simulink model "OPC_UA_daniel"  (R2024b)
settings: Solver=FixedStepAuto  StartTime=0.0  StopTime=inf  FixedStep=0.01  RelTol=1e-3
libraries: opcualib x1
settings Model: Creator=Are-Laptop  LastModifiedBy=Are-Laptop

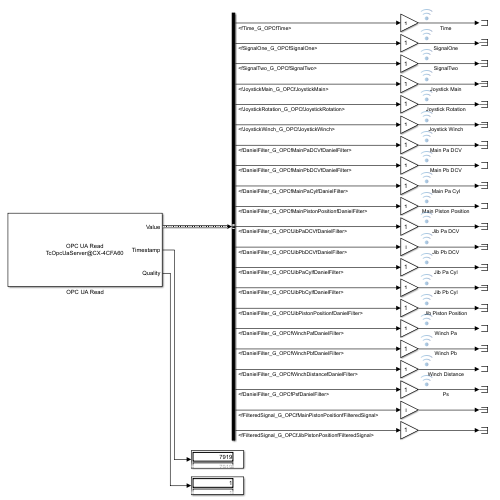
[thumbnail: Simulink's stored preview of the top-level diagram]
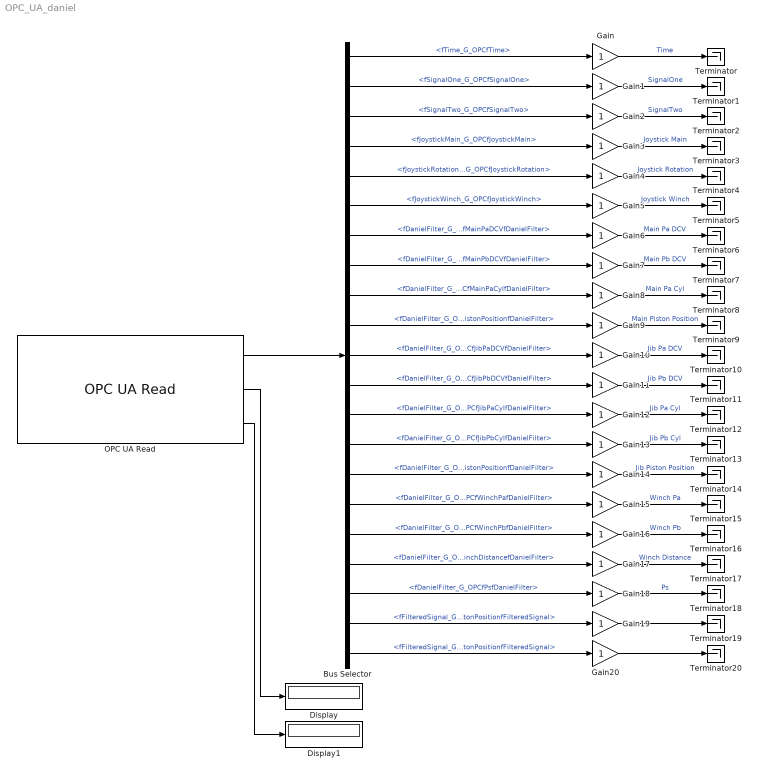
== system OPC_UA_daniel ==
  Bus Selector : BusSelector  OutputSignals=fTime_G_OPCfTime,fSignalOne_G_OPCfSignalOne,fSignalTwo_G_OPCfSignalTwo,fJoystickMain_G_OPCfJoystickMain,fJoystickRotation_G_OPCfJoystickRotation,fJoystickWinch_G_OPCfJoystickWinch,fDanielFilter_G_OPCfMainPaDCVfDanielFilter,fDanielFilter_G_OPCfMainPbDCVfDanielFilter,fDanielFilter_G_OPCfMainPaCylfDanielFilter,fDanielFilter_G_OPCfMainPistonPositionfDanielFilter,fDanielFilter_G_OPCfJibPaDCVfDanielFilter,fDanielFilter_G_OPCfJibPbDCVfDanielFilter,fDanielFilter_G_OPCfJibPaCylfDanielFilter,fDanielFilter_G_OPCfJibPbCylfDanielFilter,fDanielFilter_G_OPCfJibPistonPositionfDanielFilter,fDanielFilter_G_OPCfWinchPafDanielFilter,fDanielFilter_G_OPCfWinchPbfDanielFilter,fDanielFilter_G_OPCfWinchDistancefDanielFilter,fDanielFilter_G_OPCfPsfDanielFilter,fFilteredSignal_G_OPCfMainPistonPositionfFilteredSignal,fFilteredSignal_G_OPCfJibPistonPositionfFilteredSignal
  Display : Display
  Display1 : Display
  Gain{,1..20} (21 alike) : Gain
  OPC UA Read : opcualib/OPC UA Read  SelectedServer=TcOpcUaServer@CX-4CFA60  ServerList=TcOpcUaServer@CX-4CFA60  NodeList={ '1', 'fTime', '4', 'G_OPC.fTime', '0'; '2', 'fSignalOne', '4', 'G_OPC.fSignalOne', '0'; '3', 'fSignalTwo', '4', 'G_OPC.fSignalTwo', '0'; '4', 'fSignal', '4', 'G_OPC.fMainPaDCV.fSignal', '0'; '5', 'fFilteredSignal', '4', 'G_OPC.fMainPaDCV.fFilteredSignal', '0'; '6', 'fDanielFilter', '4', 'G_OPC.fMainPaDCV.fDanielFilter', '0'; '7', 'fSignal', '4', 'G_OPC.fMainPbDCV.fSignal', '0'; '8', 'fFilteredSignal', '4', 'G_OPC.fMainPbDCV.fFilteredSignal', '0'; '9', 'fDanielFilter', '4', 'G_OPC.fMainPbDCV.fDanielFilter', '0'; '10', 'fSignal', '4', 'G_OPC.fMainPaCyl.fSignal', '0'; '11', 'fFilteredSignal', '4', 'G_OPC.fMainPaCyl.fFilteredSignal', '0'; '12', 'fDanielFilter', '4', 'G_OPC.fMainPaCyl.fDanielFilter', '0'; '13', 'fSignal', '4', 'G_OPC.fMainPistonPosition.fSignal', '0'; '14', 'fFilteredSignal', '4', 'G_OPC.fMainPistonPosition.fFilteredSignal', '0'; '15', 'fDanielFilter', '4', 'G_OPC.fMainPistonPosition.fDanielFilter', '0'; '16', 'fSignal', '4', 'G_OPC.fJibPaDCV.fSignal', '0'; '17', 'fFilteredSignal', '4', 'G_OPC.fJibPaDCV.fFilteredSignal', '0'; '18', 'fDanielFilter', '4', 'G_OPC.fJibPaDCV.fDanielFilter', '0'; '19', 'fSignal', '4', 'G_OPC.fWinchDistance.fSignal', '0'; '20', 'fFilteredSignal', '4', 'G_OPC.fWinchDistance.fFilteredSignal', '0'; '21', 'fDanielFilter', '4', 'G_OPC.fWinchDistance.fDanielFilter', '0'; '22', 'fSignal', '4', 'G_OPC.fWinchPb.fSignal', '0'; '23', 'fFilteredSignal', '4', 'G_OPC.fWinchPb.fFilteredSignal', '0'; '24', 'fDanielFilter', '4', 'G_OPC.fWinchPb.fDanielFilter', '0'; '25', 'fSignal', '4', 'G_OPC.fWinchPa.fSignal', '0'; '26', 'fFilteredSignal', '4', 'G_OPC.fWinchPa.fFilteredSignal', '0'; '27', 'fDanielFilter', '4', 'G_OPC.fWinchPa.fDanielFilter', '0'; '28', 'fSignal', '4', 'G_OPC.fJibPistonPosition.fSignal', '0'; '29', 'fFilteredSignal', '4', 'G_OPC.fJibPistonPosition.fFilteredSignal', '0'; '30', 'fDanielFilter', '4', 'G_OPC.fJibPistonPosition.fDanielFilter', '0'; '31', 'fSignal', '4', 'G_OPC.fJibPbCyl.fSignal', '0'; '32', 'fFilteredSignal', '4', 'G_OPC.fJibPbCyl.fFilteredSignal', '0'; '33', 'fDanielFilter', '4', 'G_OPC.fJibPbCyl.fDanielFilter', '0'; '34', 'fSignal', '4', 'G_OPC.fJibPaCyl.fSignal', '0'; '35', 'fFilteredSignal', '4', 'G_OPC.fJibPaCyl.fFilteredSignal', '0'; '36', 'fDanielFilter', '4', 'G_OPC.fJibPaCyl.fDanielFilter', '0'; '37', 'fSignal', '4', 'G_OPC.fJibPbDCV.fSignal', '0'; '38', 'fFilteredSignal', '4', 'G_OPC.fJibPbDCV.fFilteredSignal', '0'; '39', 'fDanielFilter', '4', 'G_OPC.fJibPbDCV.fDanielFilter', '0'; '40', 'fJoystickWinch', '4', 'G_OPC.fJoystickWinch', '0'; '41', 'fJoystickRotation', '4', 'G_OPC.fJoystickRotation', '0'; '42', 'fJoystickMain', '4', 'G_OPC.fJoystickMain', '0'; '43', 'fJoystickJib', '4', 'G_OPC.fJoystickJib', '0'; '44', 'fJoystickExtrude', '4', 'G_OPC.fJoystickExtrude', '0'; '45', 'fValveOneOutput', '4', 'G_OPC.fValveOneOutput', '0'; '46', 'fValveOneFF', '4', 'G_OPC.fValveOneFF', '0'; '47', 'fValveOnePID', '4', 'G_OPC.fValveOnePID', '0'; '48', 'fValveTwoOutput', '4', 'G_OPC.fValveTwoOutput', '0'; '49', 'fValveTwoFF', '4', 'G_OPC.fValveTwoFF', '0'; '50', 'fValveTwoPID', '4', 'G_OPC.fValveTwoPID', '0'; '51', 'fXRef', '4', 'G_OPC.fXRef', '0'; '52', 'fXDotRef', '4', 'G_OPC.fXDotRef', '0'; '53', 'fSignal', '4', 'G_OPC.fPs.fSignal', '0'; '54', 'fFilteredSignal', '4', 'G_OPC.fPs.fFilteredSignal', '0'; '55', 'fDanielFilter', '4', 'G_OPC.fPs.fDanielFilter', '0' }  ShowQualityPort=on  ShowTimestampPort=on  ShowTimestampPortAs=Seconds since start  SampleTime=-1
  Terminator{,1..20} (21 alike) : Terminator
  wires:
  OPC UA Read/1 -> Bus Selector/1
  OPC UA Read/3 -> Display1/1
  OPC UA Read/2 -> Display/1
  Bus Selector/20 -> Gain19/1  "<fFilteredSignal_G_OPCfMainPistonPositionfFilteredSignal>"
  Bus Selector/2 -> Gain1/1  "<fSignalOne_G_OPCfSignalOne>"
  Bus Selector/9 -> Gain8/1  "<fDanielFilter_G_OPCfMainPaCylfDanielFilter>"
  Bus Selector/1 -> Gain/1  "<fTime_G_OPCfTime>"
  Bus Selector/14 -> Gain13/1  "<fDanielFilter_G_OPCfJibPbCylfDanielFilter>"
  Bus Selector/4 -> Gain3/1  "<fJoystickMain_G_OPCfJoystickMain>"
  Bus Selector/17 -> Gain16/1  "<fDanielFilter_G_OPCfWinchPbfDanielFilter>"
  Bus Selector/15 -> Gain14/1  "<fDanielFilter_G_OPCfJibPistonPositionfDanielFilter>"
  Bus Selector/3 -> Gain2/1  "<fSignalTwo_G_OPCfSignalTwo>"
  Bus Selector/5 -> Gain4/1  "<fJoystickRotation_G_OPCfJoystickRotation>"
  Bus Selector/6 -> Gain5/1  "<fJoystickWinch_G_OPCfJoystickWinch>"
  Bus Selector/11 -> Gain10/1  "<fDanielFilter_G_OPCfJibPaDCVfDanielFilter>"
  Bus Selector/7 -> Gain6/1  "<fDanielFilter_G_OPCfMainPaDCVfDanielFilter>"
  Bus Selector/12 -> Gain11/1  "<fDanielFilter_G_OPCfJibPbDCVfDanielFilter>"
  Bus Selector/10 -> Gain9/1  "<fDanielFilter_G_OPCfMainPistonPositionfDanielFilter>"
  Bus Selector/8 -> Gain7/1  "<fDanielFilter_G_OPCfMainPbDCVfDanielFilter>"
  Bus Selector/13 -> Gain12/1  "<fDanielFilter_G_OPCfJibPaCylfDanielFilter>"
  Bus Selector/16 -> Gain15/1  "<fDanielFilter_G_OPCfWinchPafDanielFilter>"
  Bus Selector/18 -> Gain17/1  "<fDanielFilter_G_OPCfWinchDistancefDanielFilter>"
  Bus Selector/19 -> Gain18/1  "<fDanielFilter_G_OPCfPsfDanielFilter>"
  Bus Selector/21 -> Gain20/1  "<fFilteredSignal_G_OPCfJibPistonPositionfFilteredSignal>"
  Gain/1 -> Terminator/1  "Time"
  Gain1/1 -> Terminator1/1  "SignalOne"
  Gain2/1 -> Terminator2/1  "SignalTwo"
  Gain3/1 -> Terminator3/1  "Joystick Main"
  Gain4/1 -> Terminator4/1  "Joystick Rotation"
  Gain5/1 -> Terminator5/1  "Joystick Winch"
  Gain6/1 -> Terminator6/1  "Main Pa DCV"
  Gain7/1 -> Terminator7/1  "Main Pb DCV"
  Gain8/1 -> Terminator8/1  "Main Pa Cyl"
  Gain9/1 -> Terminator9/1  "Main Piston Position"
  Gain10/1 -> Terminator10/1  "Jib Pa DCV"
  Gain11/1 -> Terminator11/1  "Jib Pb DCV"
  Gain12/1 -> Terminator12/1  "Jib Pa Cyl"
  Gain13/1 -> Terminator13/1  "Jib Pb Cyl"
  Gain14/1 -> Terminator14/1  "Jib Piston Position"
  Gain15/1 -> Terminator15/1  "Winch Pa"
  Gain16/1 -> Terminator16/1  "Winch Pb"
  Gain17/1 -> Terminator17/1  "Winch Distance"
  Gain18/1 -> Terminator18/1  "Ps"
  Gain19/1 -> Terminator19/1
  Gain20/1 -> Terminator20/1
